simulink model "LQR_discrete"  (R2024b)
settings: Solver=ode45  StartTime=0.0  StopTime=tsim  RelTol=1e-3  EnableMultiTasking=on
values from neighbouring files (symbols this model uses):
  C_state = eye(12)    [main.m]
  D_state = zeros(12, 1)    [main.m]
  Ts = 0.1    [main.m]    (also in point7.m)
  Ubar_z = inv(dcgain(Gz))*Ybar    [main.m]
  umax = +15    (= 15)    [main.m]
  umin = -15    [main.m]
  x0 = [3,0,3,0,3,0,3,0,3,0,3,0]    [main.m]
  Xbar_z = (eye(12) - Az) \ (Bz * Ubar_z)    [main.m]
undefined symbols (not defined in the file or in its folder): Az, Bz, Cz, K_z
settings Model: Creator=Administrator  LastModifiedBy=faiol
settings SolverCC: AlgebraicLoopSolver=TrustRegion
settings DataIOCC: LimitDataPoints=on  SaveFormat=Array  SignalLoggingSaveFormat=ModelDataLogs  ReturnWorkspaceOutputs=off
settings OptimizationCC: ExpressionDepthLimit=2147483647  InitFltsAndDblsToZero=on  LifeSpan=inf
settings DebuggingCC: UnderspecifiedInitializationDetection=Classic  MergeDetectMultiDrivingBlocksExec=none  SolverPrmCheckMsg=warning  FcnCallInpInsideContextMsg=warning  UnconnectedInputMsg=warning  UnconnectedOutputMsg=warning  UnconnectedLineMsg=warning  StateNameClashWarn=warning  SFUnexpectedBacktrackingDiag=warning  SFNoUnconditionalDefaultTransitionDiag=warning  SFExecutionAtInitializationDiag=none  ArithmeticOperatorsInVariantConditions=warning
settings HardwareCC: ProdBitPerPointer=32  ProdBitPerSizeT=32  ProdBitPerPtrDiffT=32  ProdLargestAtomicFloat=None  ProdIntDivRoundTo=Undefined  ProdEndianess=Unspecified  ProdWordSize=32  ProdHWDeviceType=32-bit Generic
settings ModelReferenceCC: EnableRefExpFcnMdlSchedulingChecks=on  PropagateSignalLabelsOutOfModel=off
settings SFSimCC: SimUseLocalCustomCode=off  CustomCodeUndefinedFunction=UseInterfaceOnly
settings RTWCC: RTWUseLocalCustomCode=off  GPUComputeCapability=3.5  DLArmComputeVersion=19.05
settings CodeAppCC: StateflowObjectComments=on
settings GRTTargetCC: TargetLangStandard=C89/C90 (ANSI)  CombineOutputUpdateFcns=off  GRTInterface=on
settings ConfigComp: CovMetricSettings=dw  CovSaveCumulativeToWorkspaceVar=on  CovSaveSingleToWorkspaceVar=on  CovExternalEMLEnable=off  CovSFcnEnable=off

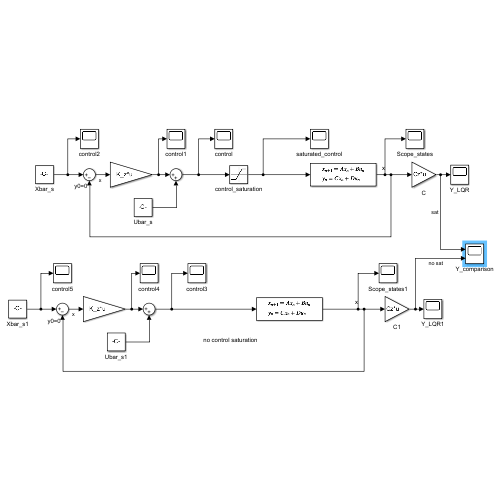
[thumbnail: Simulink's stored preview of the top-level diagram]
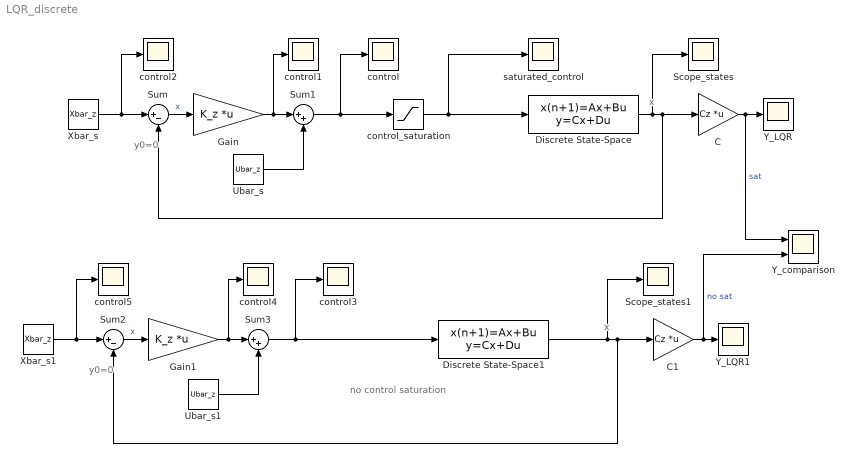
== system LQR_discrete ==
  note: no control saturation
  note: y0=0
  note: x
  note: y0=0
  note: x
  C : Gain  Gain=Cz  Multiplication=Matrix(K*u)
  C1 : Gain  Gain=Cz  Multiplication=Matrix(K*u)
  Discrete State-Space : DiscreteStateSpace  A=Az  B=Bz  C=C_state  D=D_state  InitialCondition=x0  SampleTime=Ts
  Discrete State-Space1 : DiscreteStateSpace  A=Az  B=Bz  C=C_state  D=D_state  InitialCondition=x0  SampleTime=Ts
  Gain : Gain  Gain=K_z  Multiplication=Matrix(K*u)
  Gain1 : Gain  Gain=K_z  Multiplication=Matrix(K*u)
  Scope_states : Scope
  Scope_states1 : Scope
  Sum : Sum  Inputs=|+-
  Sum1 : Sum  Inputs=|++
  Sum2 : Sum  Inputs=|+-
  Sum3 : Sum  Inputs=|++
  Ubar_s : Constant  Value=Ubar_z  SampleTime=Ts
  Ubar_s1 : Constant  Value=Ubar_z  SampleTime=Ts
  Xbar_s : Constant  Value=Xbar_z  SampleTime=Ts
  Xbar_s1 : Constant  Value=Xbar_z  SampleTime=Ts
  Y_LQR : Scope
  Y_LQR1 : Scope
  Y_comparison : Scope  NumInputPorts=2
  control{,1..5} (6 alike) : Scope
  control_saturation : Saturate  UpperLimit=umax  LowerLimit=umin
  saturated_control : Scope
  wires:
  control_saturation/1 -> Discrete State-Space/1, saturated_control/1
  Sum/1 -> Gain/1  "x"
  C/1 -> Y_comparison/1, Y_LQR/1  "sat"
  Discrete State-Space/1 -> C/1, Sum/2, Scope_states/1
  Xbar_s/1 -> control2/1, Sum/1
  Sum1/1 -> control/1, control_saturation/1
  Ubar_s/1 -> Sum1/2
  Gain/1 -> control1/1, Sum1/1
  Xbar_s1/1 -> control5/1, Sum2/1
  Sum3/1 -> Discrete State-Space1/1, control3/1
  Discrete State-Space1/1 -> C1/1, Sum2/2, Scope_states1/1
  Ubar_s1/1 -> Sum3/2
  Gain1/1 -> control4/1, Sum3/1
  Sum2/1 -> Gain1/1  "x"
  C1/1 -> Y_comparison/2, Y_LQR1/1  "no sat"
